simulink model "CONTROLLO_DINAMICA_INVERSA"  (R2022b)
settings: Solver=VariableStepAuto  StartTime=0.0  StopTime=70.0  RelTol=1e-3
undefined symbols (not defined in the file): a1, a2, d0, DiscIntNeverNeededParam, q0
settings Model: Creator=tehen  LastModifiedBy=salvatoregranata
settings OptimizationCC: ReuseModelBlockBuffer=on

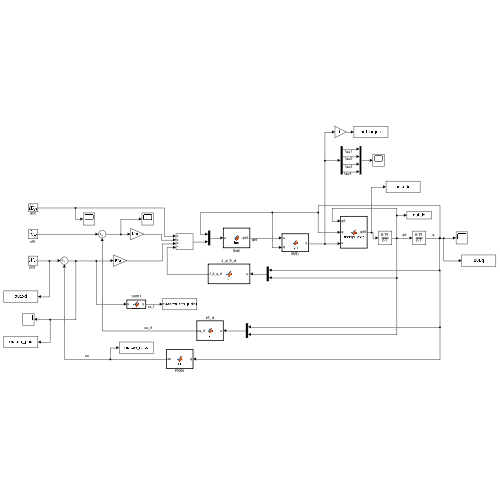
[thumbnail: Simulink's stored preview of the top-level diagram]
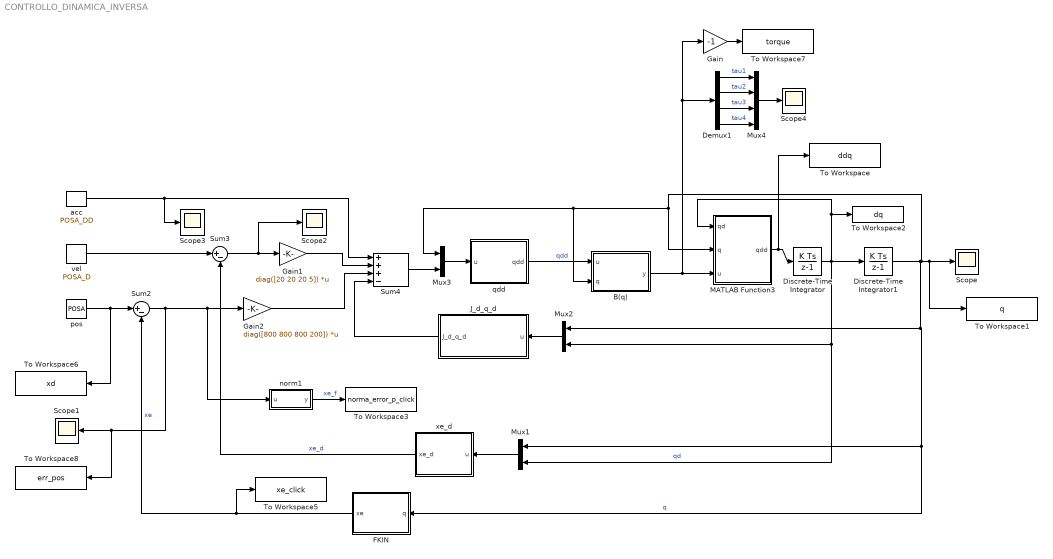
== system CONTROLLO_DINAMICA_INVERSA ==
  B(q) : MATLAB Function  TreatAsAtomicUnit=on
  Demux1 : Demux
  Discrete-Time Integrator : DiscreteIntegrator  InitialCondition=zeros(1,4)  SampleTime=1e-3  ICPrevOutput=DiscIntNeverNeededParam  ICPrevScaledInput=DiscIntNeverNeededParam
  Discrete-Time Integrator1 : DiscreteIntegrator  InitialCondition=q0  SampleTime=1e-3  ICPrevOutput=DiscIntNeverNeededParam  ICPrevScaledInput=DiscIntNeverNeededParam
  FKIN : MATLAB Function  TreatAsAtomicUnit=on
  Gain : Gain  Gain=-1
  Gain1 : Gain  Gain=diag([20 20 20 5])  Multiplication=Matrix(K*u)
  Gain2 : Gain  Gain=diag([800 800 800 200])  Multiplication=Matrix(K*u)
  J_d_q_d : MATLAB Function  TreatAsAtomicUnit=on
  MATLAB Function3 : MATLAB Function  TreatAsAtomicUnit=on
  Mux1 : Mux  Inputs=2
  Mux2 : Mux  Inputs=2
  Mux3 : Mux  Inputs=2
  Mux4 : Mux
  Scope{,1..4} (5 alike) : Scope
  Sum2 : Sum  Inputs=|+-
  Sum3 : Sum  Inputs=|+-
  Sum4 : Sum  Inputs=+++-
  To Workspace : ToWorkspace  VariableName=ddq  SaveFormat=Timeseries  SampleTime=-1
  To Workspace1 : ToWorkspace  VariableName=q  SaveFormat=Structure With Time  SampleTime=-1
  To Workspace2 : ToWorkspace  VariableName=dq  SaveFormat=Structure With Time  SampleTime=-1
  To Workspace3 : ToWorkspace  VariableName=norma_error_p_click  SaveFormat=Timeseries  SampleTime=-1
  To Workspace5 : ToWorkspace  VariableName=xe_click  SaveFormat=Timeseries  SampleTime=-1
  To Workspace6 : ToWorkspace  VariableName=xd  SaveFormat=Timeseries  SampleTime=-1
  To Workspace7 : ToWorkspace  VariableName=torque  SaveFormat=Structure With Time  SampleTime=-1
  To Workspace8 : ToWorkspace  VariableName=err_pos  SaveFormat=Structure With Time  SampleTime=-1
  acc : FromWorkspace  VariableName=POSA_DD  SampleTime=0.001
      mask Display: image('/Users/salvatoregranata/Desktop/TESINA_FR_APICELLA_GIORDANO 2/Foto/Screenshot 2023-07-28 alle 15.02.35.png'); % Use "Edit Image" on toolstrip to change.
  norm1 : MATLAB Function  TreatAsAtomicUnit=on
  "pos " : FromWorkspace  VariableName=POSA  SampleTime=0.001
      mask Display: image('/Users/salvatoregranata/Desktop/TESINA_FR_APICELLA_GIORDANO 2/Foto/Screenshot 2023-07-27 alle 22.18.08 copia.png'); % Use "Edit Image" on toolstrip to change.
  qdd : MATLAB Function  TreatAsAtomicUnit=on
  "vel " : FromWorkspace  VariableName=POSA_D  SampleTime=0.001
      mask Display: image('/Users/salvatoregranata/Desktop/TESINA_FR_APICELLA_GIORDANO 2/Foto/Screenshot 2023-07-27 alle 22.16.25.png'); % Use "Edit Image" on toolstrip to change.
  xe_d : MATLAB Function  TreatAsAtomicUnit=on
  wires:
  FKIN/1(xe) -> Sum2/2, To Workspace5/1  "xe"
  Discrete-Time Integrator1/1 -> To Workspace1/1, Scope/1, MATLAB Function3/2(q), B(q)/2(q), Mux3/1, Mux2/1, Mux1/1, FKIN/1(q)  "q"
  Mux2/1 -> J_d_q_d/1(u)
  Discrete-Time Integrator/1 -> Discrete-Time Integrator1/1, MATLAB Function3/1(qd), To Workspace2/1, Mux1/2, Mux2/2  "qd"
  Mux3/1 -> qdd/1(u)
  Gain1/1 -> Sum4/2
  Gain2/1 -> Sum4/3
  xe_d/1(xe_d) -> Sum3/2  "xe_d"
  qdd/1(qdd) -> B(q)/1(u)  "qdd"
  Sum3/1 -> Scope2/1, Gain1/1
  J_d_q_d/1(J_d_q_d) -> Sum4/4
  "vel "/1 -> Sum3/1
  Sum2/1 -> norm1/1(u), Gain2/1, To Workspace8/1, Scope1/1
  Mux1/1 -> xe_d/1(u)
  acc/1 -> Scope3/1, Sum4/1
  "pos "/1 -> To Workspace6/1, Sum2/1
  Sum4/1 -> Mux3/2
  norm1/1(y) -> To Workspace3/1  "xe_f"
  MATLAB Function3/1(qdd) -> To Workspace/1, Discrete-Time Integrator/1
  Demux1/3 -> Mux4/3  "tau3"
  Demux1/1 -> Mux4/1  "tau1"
  Demux1/2 -> Mux4/2  "tau2"
  B(q)/1(y) -> Gain/1, Demux1/1, MATLAB Function3/3(u)
  Mux4/1 -> Scope4/1
  Demux1/4 -> Mux4/4  "tau4"
  Gain/1 -> To Workspace7/1

== matlab function CONTROLLO_DINAMICA_INVERSA/xe_d ==
  data: u input; xe_d output; a1 parameter; a2 parameter
function xe_d = fcn(u, a1, a2)

q = u(1:4);
u2 = u(5:8);

% Jacobiano
J = [ -a1*sin(q(1))-a2*sin(q(1)+q(2))   -a2*sin(q(1)+q(2))  0   0   ;
       a1*cos(q(1))+a2*cos(q(1)+q(2))    a2*cos(q(1)+q(2))  0   0   ;
                   0                              0         1   0   ;
                   1                              1         0   1   ];
               
    xe_d = J*u2;
end

== matlab function CONTROLLO_DINAMICA_INVERSA/FKIN ==
  data: q input; xe output; a2 parameter; a1 parameter; d0 parameter
function xe = fcn(q, a2, a1, d0)

theta1 = q(1);
theta2 = q(2);
d3 = q(3);
theta4 = q(4);

% Cinematica diretta
xe = [a1*cos(theta1)+a2*cos(theta1+theta2) ;
      a1*sin(theta1)+a2*sin(theta1+theta2) ;
      d3+d0 ;
      theta1+theta2+theta4; ];
end

== matlab function CONTROLLO_DINAMICA_INVERSA/qdd ==
  data: u input; qdd output; a1 parameter; a2 parameter
function qdd = fcn(u, a1, a2)

q = u(1:4);
u2 = u(5:8);

% Jacobiano
J = [ -a1*sin(q(1))-a2*sin(q(1)+q(2))   -a2*sin(q(1)+q(2))  0   0   ;
       a1*cos(q(1))+a2*cos(q(1)+q(2))    a2*cos(q(1)+q(2))  0   0   ;
                   0                              0         1   0   ;
                   1                              1         0   1   ];

% Damped Least Squares
intervallo = 0.05;
k = 0.1;

if(abs(det(J))) < intervallo;
    J = J' * inv(J*J' + eye(4)*k^2);
    qdd = J*(u2);
else
    qdd = inv(J)*(u2);
end

== matlab function CONTROLLO_DINAMICA_INVERSA/J_d_q_d ==
  data: u input; J_d_q_d output; a1 parameter; a2 parameter
function J_d_q_d = fcn(u, a1, a2)

q = u(1:4);
q1_d=u(5);
q2_d=u(6);
u2 = u(5:8);
% Jacobiano derivato
               
J_d = [ (-q1_d + q2_d)*(a2*cos(q(1)+q(2)))-q1_d*a1*cos(q(1)),  -(q1_d+q2_d)*(a2*cos(q(1)+q(2))),   0,  0;
         -(q1_d+q2_d)*(a2*sin(q(1)+q(2)))-q1_d*a1*sin(q(1)),  -(q1_d+q2_d)*(a2*sin(q(1)+q(2))),   0,  0;
         0, 0, 0, 0;
         0, 0, 0, 0;];
               
J_d_q_d = J_d*u2;
    
end

== matlab function CONTROLLO_DINAMICA_INVERSA/norm1 ==
  data: u input; y output
function y = norm(u)
y = norm(u);

== matlab function CONTROLLO_DINAMICA_INVERSA/B(q) ==
  data: u input; y output; q input
function y = fcn(u,q)

q_1=q(1);
q_2=q(2);
q_3=q(3);
q_4=q(4);

%B è ottenuta da subs(B,pigreco,param_esatti)
B=[(45*cos(q_2))/4 + 25421/1000, (45*cos(q_2))/8 + 20177/2000,  1/4, 51/50;
(45*cos(q_2))/8 + 20177/2000,                   20177/2000,  1/4, 51/50;
                         1/4,                          1/4, 45/2,     0;
                       51/50,                        51/50,    0,   7/5]; 

y=B*u;

== matlab function CONTROLLO_DINAMICA_INVERSA/MATLAB Function3 ==
  data: qd input; q input; u input; qdd output
function qdd = manipulator(qd, q, u)

q_1 = q(1);
q_2 = q(2);
q_3 = q(3);
q_4 = q(4);
qd_1 = qd(1);
qd_2 = qd(2);
qd_3 = qd(3);
qd_4 = qd(4);

   
n = [ qd_1/10000 - (51*qd_1*qd_2*sin(q_2))/8 - (qd_2*sin(q_2)*(51*qd_1 + 51*qd_2))/8;
                                                 (51*sin(q_2)*qd_1^2)/8 + qd_2/10000;
                                                                  4*qd_3 + 12753/100;
                                                                              2*qd_4];
 
                                                                    
B = [ (51*cos(q_2))/4 + 26921/1000, (51*cos(q_2))/8 + 21677/2000,  1/4, 51/50;
      (51*cos(q_2))/8 + 21677/2000,                   21677/2000,  1/4, 51/50;
                               1/4,                          1/4, 51/2,     0;
                             51/50,                        51/50,    0,   7/5];
 
qdd = inv(B)*(u-n);
